simulink model "gpio_bidir"  (R2016b)
settings: Solver=VariableStepAuto  StartTime=0.0  StopTime=10.0  RelTol=1e-3
libraries: xbsIndex_r4 x7
settings Model: Creator=qwerty40  LastModifiedBy=qwerty40

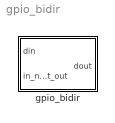
== system gpio_bidir ==
  gpio_bidir : Subsystem  Tag=xps:gpio_bidir  mask(gpio_bidir){io_group=gpio, bitwidth=4, bit_index=[0, 1, 2, 3]}
      mask prompts: io_group "I/O group"; bitwidth "Data bitwidth"; bit_index "GPIO bit index"
      mask help: Bi-directional GPIO interface.
      mask init:
      | gpio_bidir_mask;
      mask Help:
      | Inputs:
      | - din: data input (size set by Data bitwidth parameter in bits)
      | - in_not_out: The control signal, 1 for input and 0 for output.
      | 
      | Outputs:
      | - dout: The data output
      | 
      | When using bitwidths greater than one, you should specify a vector of bit indices to use. GPIO bit index should have the same number of elements as the I/O bitwidth.
      | 
      | See below for GPIO (GPIO bit indices correspond to TEST#):
      | 
      | Example: If you set Data bitwidth to 4, you might want you use GPIO bit indices [0, 1, 2, 3].
      | 
      | SNAP board
      | gpio:
      |     iostd: LVCMOS25
      |     loc:
      |       - B21 (TEST0)
      |       - C21 (TEST1)
      |       - B20 (TEST2)
      |       - A20 (TEST3)
      |       - H24 (TEST4)
      |       - H23 (TEST5)
      |       - B26 (TEST6)
      |       - R25 (TEST7)
      |       - L17 (TEST8)
      |       - K18 (TEST9)
      | led:
      |     iostd: LVCMOS25
      |     loc:
      |       - C13
      |       - C14
      |       - D13
      |       - D14
      |       - E12
      |       - E13
      mask TypeOptions io_group: led | gpio | sync_in | sync_out | zdok0 | zdok1

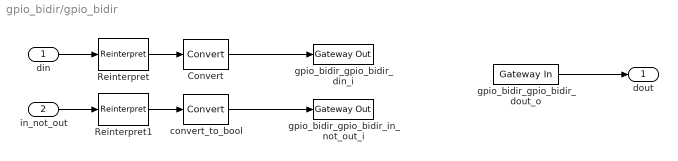
== system gpio_bidir/gpio_bidir ==
  din : Inport
  in_not_out : Inport  Port=2
  Convert : xbsIndex_r4/Convert  gui_display_data_type=Fixed-point  arith_type=Unsigned  n_bits=4  bin_pt=0  float_type=Single  exp_bits=8  fraction_bits=24  quantization=Truncate  overflow=Wrap  en=off  latency=1  pipeline=off  dbl_ovrd=off  block_type=convert
  Reinterpret : xbsIndex_r4/Reinterpret  force_arith_type=on  arith_type=Unsigned  force_bin_pt=on  bin_pt=0  block_type=reinterpret
  Reinterpret1 : xbsIndex_r4/Reinterpret  force_arith_type=on  arith_type=Unsigned  force_bin_pt=on  bin_pt=0  block_type=reinterpret
  convert_to_bool : xbsIndex_r4/Convert  gui_display_data_type=Boolean  arith_type=Boolean  n_bits=16  bin_pt=14  float_type=Single  exp_bits=8  fraction_bits=24  quantization=Truncate  overflow=Wrap  en=off  latency=1  pipeline=off  dbl_ovrd=off  block_type=convert
  gpio_bidir_gpio_bidir_din_i : xbsIndex_r4/Gateway Out  inherit_from_input=off  hdl_port=on  rows=1  columns=1  UseAsDAC=off  DACChannel='1'  interface=None  automatic_assignment=on  address_offset=hex2dec('00')  intf_name=''  intf_description=''  timing_constraint=None  locs_specified=off  LOCs={}  io_standard={}  block_type=gatewayout
  gpio_bidir_gpio_bidir_dout_o : xbsIndex_r4/Gateway In  gui_display_data_type=Fixed-point  arith_type=Unsigned  n_bits=4  bin_pt=0  preci_type=Single  exp_width=8  frac_width=24  rows=1  columns=1  quantization=Truncate  overflow=Wrap  period=1  UseAsADC=off  ADCChannel='1'  interface=None  automatic_assignment=on  address_offset=hex2dec('00')  intf_name=''  intf_description=''  default_value=0  timing_constraint=None  locs_specified=off  LOCs={}  io_standard={}  inherit_from_input=off  hdl_port=on  dbl_ovrd=off  block_type=gatewayin
  gpio_bidir_gpio_bidir_in_not_out_i : xbsIndex_r4/Gateway Out  inherit_from_input=off  hdl_port=on  rows=1  columns=1  UseAsDAC=off  DACChannel='1'  interface=None  automatic_assignment=on  address_offset=hex2dec('00')  intf_name=''  intf_description=''  timing_constraint=None  locs_specified=off  LOCs={}  io_standard={}  block_type=gatewayout
  dout : Outport
  wires:
  in_not_out/1 -> Reinterpret1/1
  din/1 -> Reinterpret/1
  Reinterpret/1 -> Convert/1
  Reinterpret1/1 -> convert_to_bool/1
  Convert/1 -> gpio_bidir_gpio_bidir_din_i/1
  convert_to_bool/1 -> gpio_bidir_gpio_bidir_in_not_out_i/1
  gpio_bidir_gpio_bidir_dout_o/1 -> dout/1
